simulink model "multi_vehicle"  (R2024a)
settings: Solver=VariableStepAuto  StartTime=0.0  StopTime=600  RelTol=1e-3
settings Model: Creator=sprinkle  LastModifiedBy=Yizhou
settings OptimizationCC: ReuseModelBlockBuffer=off
settings RTWCC: GPUComputeCapability=3.5

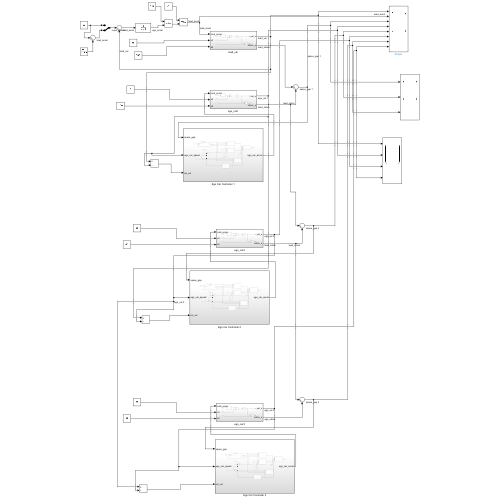
[thumbnail: Simulink's stored preview of the top-level diagram]
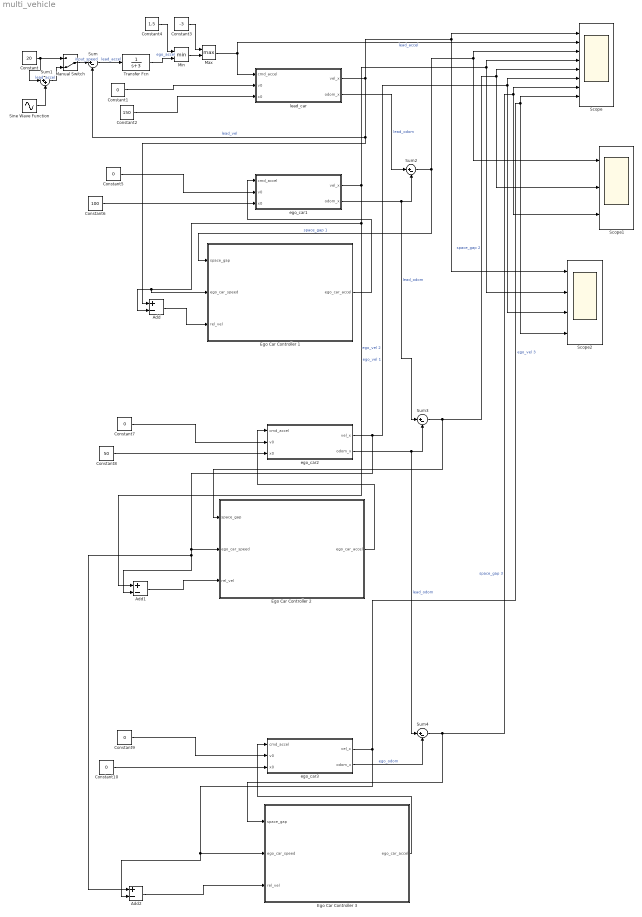
== system multi_vehicle ==
  Add : Sum  Inputs=+-
  Add1 : Sum  Inputs=+-
  Add2 : Sum  Inputs=+-
  Constant : Constant  Value=20
  Constant{1,5,7,9..10} (5 alike) : Constant  Value=0
  Constant2 : Constant  Value=150
  Constant3 : Constant  Value=-3
  Constant4 : Constant  Value=1.5
  Constant6 : Constant  Value=100
  Constant8 : Constant  Value=50
  Ego Car Controller 1 : Subsystem
  Ego Car Controller 2 : Subsystem
  Ego Car Controller 3 : Subsystem
  Manual Switch : ManualSwitch  CurrentSetting=0
  Max : MinMax  Function=max  Inputs=2
  Min : MinMax  Inputs=2
  Scope : Scope  NumInputPorts=8
  Scope1 : Scope  NumInputPorts=3
  Scope2 : Scope  NumInputPorts=4
  Sine Wave Function : Sin  Amplitude=3  Frequency=0.3  SampleTime=0
  Sum{,2..4} (4 alike) : Sum  Inputs=|+-
  Sum1 : Sum  Inputs=|++
  Transfer Fcn : TransferFcn  Denominator=[1 3]
  ego_car1 : Subsystem
  ego_car2 : Subsystem
  ego_car3 : Subsystem
  lead_car : Subsystem
  wires:
  Constant/1 -> Sum1/1, Manual Switch/1
  lead_car/1(vel_x) -> Scope2/1, Scope/1, Add/1, Sum/2  "lead_vel"
  Constant1/1 -> lead_car/2(v0)
  Constant2/1 -> lead_car/3(x0)
  Sum/1 -> Transfer Fcn/1  "lead_accel"
  Manual Switch/1 -> Sum/1  "input_speed"
  Max/1 -> lead_car/1(cmd_accel), Scope/2  "lead_accel"
  Constant4/1 -> Min/1
  Constant3/1 -> Max/1
  Min/1 -> Max/2
  Sine Wave Function/1 -> Sum1/2
  Sum1/1 -> Manual Switch/2  "lead_accel"
  Transfer Fcn/1 -> Min/2  "ego_accel"
  Sum2/1 -> Ego Car Controller 1/1(space_gap), Scope1/1, Scope/3  "space_gap 1"
  lead_car/2(odom_x) -> Sum2/1  "lead_odom"
  ego_car1/1(vel_x) -> Add1/1, Ego Car Controller 1/2(ego_car_speed), Add/2, Scope2/2, Scope/4  "ego_vel 1"
  Ego Car Controller 1/1(ego_car_accel) -> ego_car1/1(cmd_accel)
  Constant5/1 -> ego_car1/2(v0)
  Constant6/1 -> ego_car1/3(x0)
  Constant8/1 -> ego_car2/3(x0)
  Constant7/1 -> ego_car2/2(v0)
  Ego Car Controller 2/1(ego_car_accel) -> ego_car2/1(cmd_accel)
  Sum3/1 -> Ego Car Controller 2/1(space_gap), Scope1/2, Scope/5  "space_gap 2"
  ego_car1/2(odom_x) -> Sum2/2, Sum3/1  "lead_odom"
  Ego Car Controller 3/1(ego_car_accel) -> ego_car3/1(cmd_accel)
  ego_car2/1(vel_x) -> Ego Car Controller 2/2(ego_car_speed), Add1/2, Add2/1, Scope2/3, Scope/6  "ego_vel 2"
  ego_car3/1(vel_x) -> Ego Car Controller 3/2(ego_car_speed), Add2/2, Scope2/4, Scope/8  "ego_vel 3"
  ego_car3/2(odom_x) -> Sum4/2  "ego_odom"
  Constant10/1 -> ego_car3/3(x0)
  Constant9/1 -> ego_car3/2(v0)
  Sum4/1 -> Ego Car Controller 3/1(space_gap), Scope1/3, Scope/7  "space_gap 3"
  ego_car2/2(odom_x) -> Sum4/1, Sum3/2  "lead_odom"
  Add/1 -> Ego Car Controller 1/3(rel_vel)
  Add1/1 -> Ego Car Controller 2/3(rel_vel)
  Add2/1 -> Ego Car Controller 3/3(rel_vel)

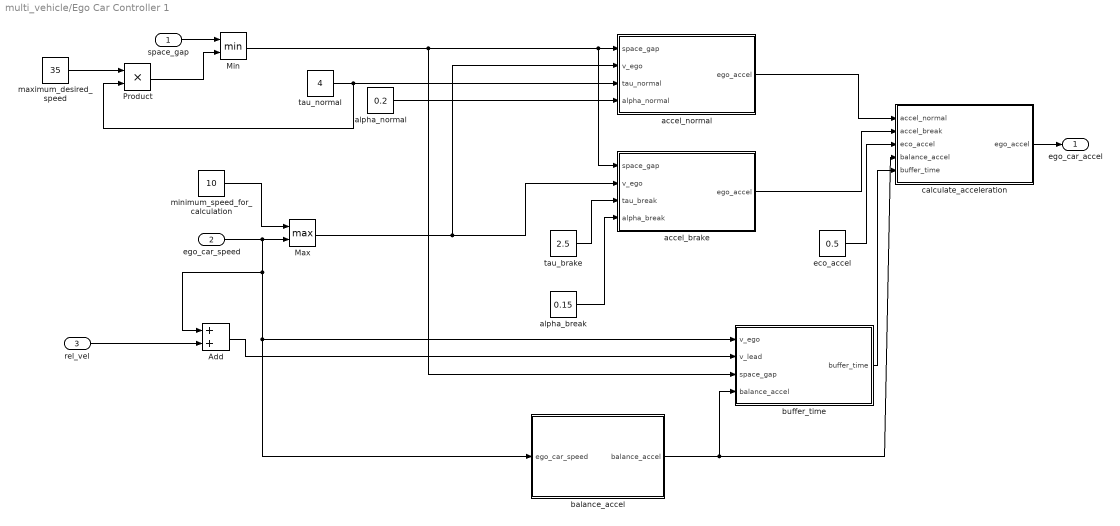
== system multi_vehicle/Ego Car Controller 1 ==
  space_gap : Inport
  ego_car_speed : Inport  Port=2
  rel_vel : Inport  Port=3
  Add : Sum
  Max : MinMax  Function=max  Inputs=2
  Min : MinMax  Inputs=2
  Product : Product
  accel_brake : MATLAB Function  TreatAsAtomicUnit=on
  accel_normal : MATLAB Function  TreatAsAtomicUnit=on
  alpha_break : Constant  Value=0.15
  alpha_normal : Constant  Value=0.2
  balance_accel : MATLAB Function  TreatAsAtomicUnit=on
  buffer_time : MATLAB Function  TreatAsAtomicUnit=on
  calculate_acceleration : MATLAB Function  TreatAsAtomicUnit=on
  eco_accel : Constant  Value=0.5
  maximum_desired_speed : Constant  Value=35
  minimum_speed_for_calculation : Constant  Value=10
  tau_brake : Constant  Value=2.5
  tau_normal : Constant  Value=4
  ego_car_accel : Outport
  wires:
  Max/1 -> accel_normal/2(v_ego), accel_brake/2(v_ego)
  Min/1 -> buffer_time/3(space_gap), accel_normal/1(space_gap), accel_brake/1(space_gap)
  alpha_normal/1 -> accel_normal/4(alpha_normal)
  tau_brake/1 -> accel_brake/3(tau_break)
  alpha_break/1 -> accel_brake/4(alpha_break)
  accel_normal/1(ego_accel) -> calculate_acceleration/1(accel_normal)
  eco_accel/1 -> calculate_acceleration/3(eco_accel)
  balance_accel/1(balance_accel) -> buffer_time/4(balance_accel), calculate_acceleration/4(balance_accel)
  accel_brake/1(ego_accel) -> calculate_acceleration/2(accel_break)
  ego_car_speed/1 -> Add/1, buffer_time/1(v_ego), balance_accel/1(ego_car_speed), Max/2
  minimum_speed_for_calculation/1 -> Max/1
  space_gap/1 -> Min/1
  Product/1 -> Min/2
  calculate_acceleration/1(ego_accel) -> ego_car_accel/1
  tau_normal/1 -> Product/2, accel_normal/3(tau_normal)
  maximum_desired_speed/1 -> Product/1
  rel_vel/1 -> Add/2
  buffer_time/1(buffer_time) -> calculate_acceleration/5(buffer_time)
  Add/1 -> buffer_time/2(v_lead)

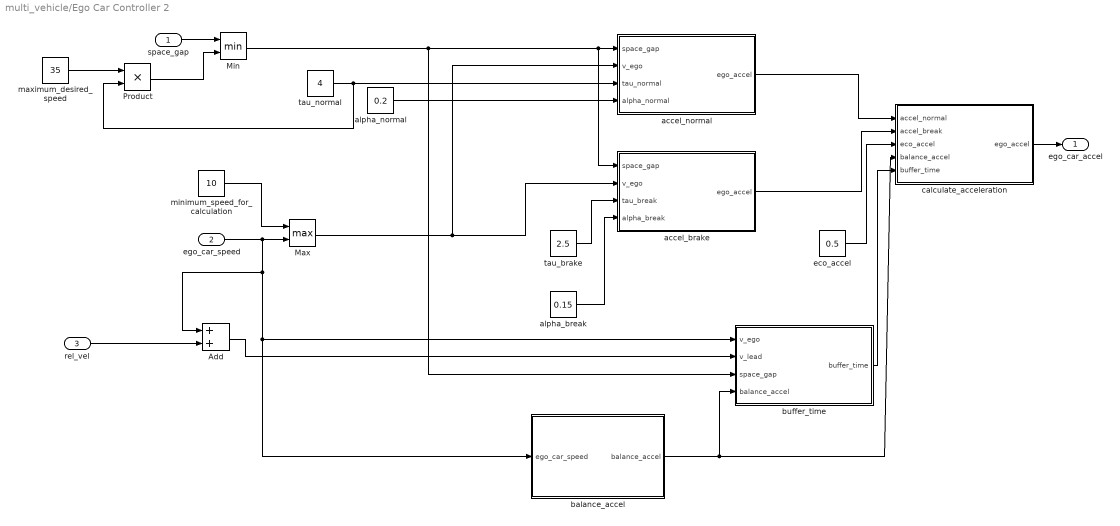
== system multi_vehicle/Ego Car Controller 2 ==
  space_gap : Inport
  ego_car_speed : Inport  Port=2
  rel_vel : Inport  Port=3
  Add : Sum
  Max : MinMax  Function=max  Inputs=2
  Min : MinMax  Inputs=2
  Product : Product
  accel_brake : MATLAB Function  TreatAsAtomicUnit=on
  accel_normal : MATLAB Function  TreatAsAtomicUnit=on
  alpha_break : Constant  Value=0.15
  alpha_normal : Constant  Value=0.2
  balance_accel : MATLAB Function  TreatAsAtomicUnit=on
  buffer_time : MATLAB Function  TreatAsAtomicUnit=on
  calculate_acceleration : MATLAB Function  TreatAsAtomicUnit=on
  eco_accel : Constant  Value=0.5
  maximum_desired_speed : Constant  Value=35
  minimum_speed_for_calculation : Constant  Value=10
  tau_brake : Constant  Value=2.5
  tau_normal : Constant  Value=4
  ego_car_accel : Outport
  wires:
  Max/1 -> accel_normal/2(v_ego), accel_brake/2(v_ego)
  Min/1 -> buffer_time/3(space_gap), accel_normal/1(space_gap), accel_brake/1(space_gap)
  alpha_normal/1 -> accel_normal/4(alpha_normal)
  tau_brake/1 -> accel_brake/3(tau_break)
  alpha_break/1 -> accel_brake/4(alpha_break)
  accel_normal/1(ego_accel) -> calculate_acceleration/1(accel_normal)
  eco_accel/1 -> calculate_acceleration/3(eco_accel)
  balance_accel/1(balance_accel) -> buffer_time/4(balance_accel), calculate_acceleration/4(balance_accel)
  accel_brake/1(ego_accel) -> calculate_acceleration/2(accel_break)
  ego_car_speed/1 -> Add/1, buffer_time/1(v_ego), balance_accel/1(ego_car_speed), Max/2
  minimum_speed_for_calculation/1 -> Max/1
  space_gap/1 -> Min/1
  Product/1 -> Min/2
  calculate_acceleration/1(ego_accel) -> ego_car_accel/1
  tau_normal/1 -> Product/2, accel_normal/3(tau_normal)
  maximum_desired_speed/1 -> Product/1
  rel_vel/1 -> Add/2
  buffer_time/1(buffer_time) -> calculate_acceleration/5(buffer_time)
  Add/1 -> buffer_time/2(v_lead)

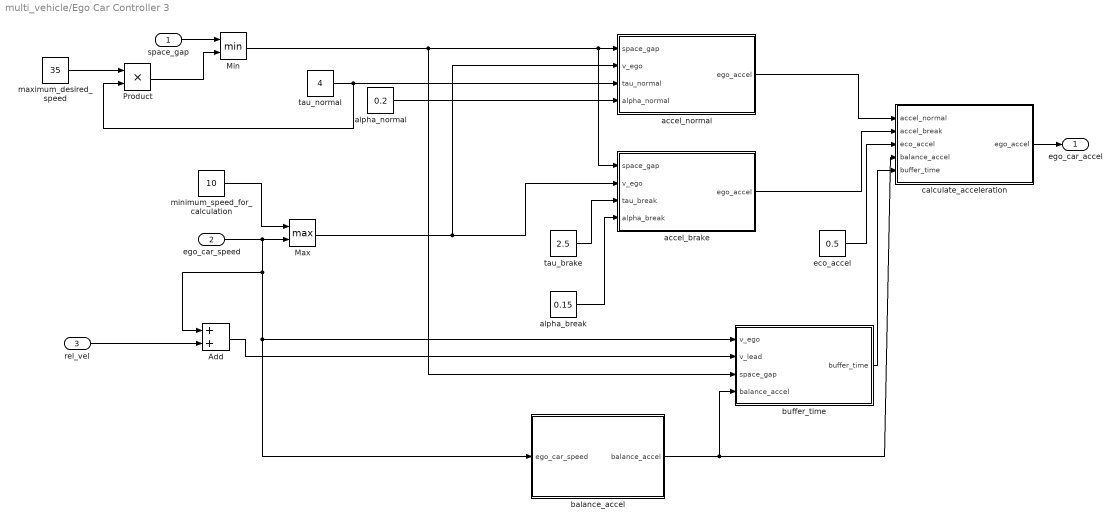
== system multi_vehicle/Ego Car Controller 3 ==
  space_gap : Inport
  ego_car_speed : Inport  Port=2
  rel_vel : Inport  Port=3
  Add : Sum
  Max : MinMax  Function=max  Inputs=2
  Min : MinMax  Inputs=2
  Product : Product
  accel_brake : MATLAB Function  TreatAsAtomicUnit=on
  accel_normal : MATLAB Function  TreatAsAtomicUnit=on
  alpha_break : Constant  Value=0.15
  alpha_normal : Constant  Value=0.2
  balance_accel : MATLAB Function  TreatAsAtomicUnit=on
  buffer_time : MATLAB Function  TreatAsAtomicUnit=on
  calculate_acceleration : MATLAB Function  TreatAsAtomicUnit=on
  eco_accel : Constant  Value=0.5
  maximum_desired_speed : Constant  Value=35
  minimum_speed_for_calculation : Constant  Value=10
  tau_brake : Constant  Value=2.5
  tau_normal : Constant  Value=4
  ego_car_accel : Outport
  wires:
  Max/1 -> accel_normal/2(v_ego), accel_brake/2(v_ego)
  Min/1 -> buffer_time/3(space_gap), accel_normal/1(space_gap), accel_brake/1(space_gap)
  alpha_normal/1 -> accel_normal/4(alpha_normal)
  tau_brake/1 -> accel_brake/3(tau_break)
  alpha_break/1 -> accel_brake/4(alpha_break)
  accel_normal/1(ego_accel) -> calculate_acceleration/1(accel_normal)
  eco_accel/1 -> calculate_acceleration/3(eco_accel)
  balance_accel/1(balance_accel) -> buffer_time/4(balance_accel), calculate_acceleration/4(balance_accel)
  accel_brake/1(ego_accel) -> calculate_acceleration/2(accel_break)
  ego_car_speed/1 -> Add/1, buffer_time/1(v_ego), balance_accel/1(ego_car_speed), Max/2
  minimum_speed_for_calculation/1 -> Max/1
  space_gap/1 -> Min/1
  Product/1 -> Min/2
  calculate_acceleration/1(ego_accel) -> ego_car_accel/1
  tau_normal/1 -> Product/2, accel_normal/3(tau_normal)
  maximum_desired_speed/1 -> Product/1
  rel_vel/1 -> Add/2
  buffer_time/1(buffer_time) -> calculate_acceleration/5(buffer_time)
  Add/1 -> buffer_time/2(v_lead)

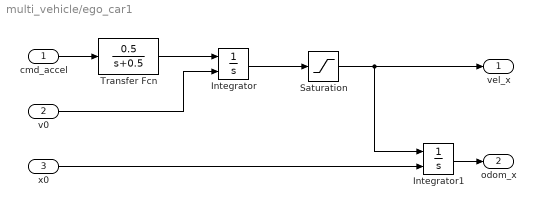
== system multi_vehicle/ego_car1 ==
  cmd_accel : Inport
  v0 : Inport  Port=2
  x0 : Inport  Port=3
  Integrator : Integrator  InitialConditionSource=external
  Integrator1 : Integrator  InitialConditionSource=external
  Saturation : Saturate  UpperLimit=80  LowerLimit=0
  Transfer Fcn : TransferFcn  Numerator=[0.5]  Denominator=[1 0.5]
  vel_x : Outport
  odom_x : Outport  Port=2
  wires:
  v0/1 -> Integrator/2
  cmd_accel/1 -> Transfer Fcn/1
  Transfer Fcn/1 -> Integrator/1
  Integrator1/1 -> odom_x/1
  Integrator/1 -> Saturation/1
  x0/1 -> Integrator1/2
  Saturation/1 -> vel_x/1, Integrator1/1

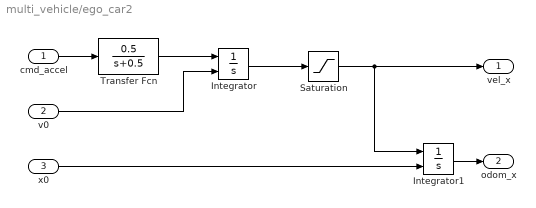
== system multi_vehicle/ego_car2 ==
  cmd_accel : Inport
  v0 : Inport  Port=2
  x0 : Inport  Port=3
  Integrator : Integrator  InitialConditionSource=external
  Integrator1 : Integrator  InitialConditionSource=external
  Saturation : Saturate  UpperLimit=80  LowerLimit=0
  Transfer Fcn : TransferFcn  Numerator=[0.5]  Denominator=[1 0.5]
  vel_x : Outport
  odom_x : Outport  Port=2
  wires:
  v0/1 -> Integrator/2
  cmd_accel/1 -> Transfer Fcn/1
  Transfer Fcn/1 -> Integrator/1
  Integrator1/1 -> odom_x/1
  Integrator/1 -> Saturation/1
  x0/1 -> Integrator1/2
  Saturation/1 -> vel_x/1, Integrator1/1

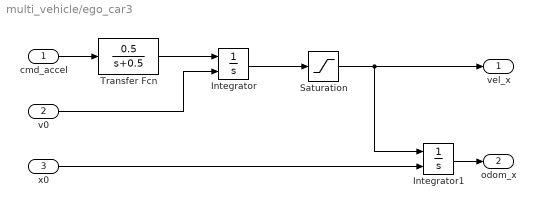
== system multi_vehicle/ego_car3 ==
  cmd_accel : Inport
  v0 : Inport  Port=2
  x0 : Inport  Port=3
  Integrator : Integrator  InitialConditionSource=external
  Integrator1 : Integrator  InitialConditionSource=external
  Saturation : Saturate  UpperLimit=80  LowerLimit=0
  Transfer Fcn : TransferFcn  Numerator=[0.5]  Denominator=[1 0.5]
  vel_x : Outport
  odom_x : Outport  Port=2
  wires:
  v0/1 -> Integrator/2
  cmd_accel/1 -> Transfer Fcn/1
  Transfer Fcn/1 -> Integrator/1
  Integrator1/1 -> odom_x/1
  Integrator/1 -> Saturation/1
  x0/1 -> Integrator1/2
  Saturation/1 -> vel_x/1, Integrator1/1

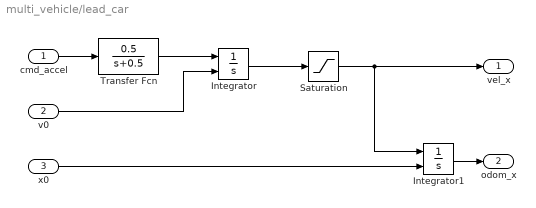
== system multi_vehicle/lead_car ==
  cmd_accel : Inport
  v0 : Inport  Port=2
  x0 : Inport  Port=3
  Integrator : Integrator  InitialConditionSource=external
  Integrator1 : Integrator  InitialConditionSource=external
  Saturation : Saturate  UpperLimit=80  LowerLimit=0
  Transfer Fcn : TransferFcn  Numerator=[0.5]  Denominator=[1 0.5]
  vel_x : Outport
  odom_x : Outport  Port=2
  wires:
  v0/1 -> Integrator/2
  cmd_accel/1 -> Transfer Fcn/1
  Transfer Fcn/1 -> Integrator/1
  Integrator1/1 -> odom_x/1
  Integrator/1 -> Saturation/1
  x0/1 -> Integrator1/2
  Saturation/1 -> vel_x/1, Integrator1/1

== matlab function multi_vehicle/Ego Car Controller 3/accel_brake ==
  data: space_gap input; ego_accel output; v_ego input; tau_break input; alpha_break input
function ego_accel = fcn(space_gap, v_ego, tau_break, alpha_break)

ego_accel = (alpha_break*(space_gap - tau_break * v_ego));
ego_accel = min(ego_accel, 1.5);
ego_accel = max(ego_accel, -3);

== matlab function multi_vehicle/Ego Car Controller 3/accel_normal ==
  data: space_gap input; v_ego input; tau_normal input; alpha_normal input; ego_accel output
function ego_accel = fcn(space_gap, v_ego, tau_normal, alpha_normal)

ego_accel = (alpha_normal * (space_gap - tau_normal * v_ego));
ego_accel = min(ego_accel, 1.5);
ego_accel = max(ego_accel, -3);

== matlab function multi_vehicle/Ego Car Controller 1/accel_normal ==
  data: space_gap input; v_ego input; tau_normal input; alpha_normal input; ego_accel output
function ego_accel = fcn(space_gap, v_ego, tau_normal, alpha_normal)

ego_accel = (alpha_normal * (space_gap - tau_normal * v_ego));
ego_accel = min(ego_accel, 1.5);
ego_accel = max(ego_accel, -3);

== matlab function multi_vehicle/Ego Car Controller 3/balance_accel ==
  data: ego_car_speed input; balance_accel output
function balance_accel = fcn(ego_car_speed)

balance_accel = -0.00021453 * (ego_car_speed * ego_car_speed) - 0.14715;

== matlab function multi_vehicle/Ego Car Controller 3/buffer_time ==
  data: v_ego input; v_lead input; space_gap input; buffer_time output; balance_accel input
function buffer_time = fcn(v_ego, v_lead, space_gap, balance_accel)

% Calculate distance needed for ego car to match lead_car speed to brake at
% balance_accel
brake_dist = (v_ego+v_lead)/2*(v_ego - v_lead)/(0-balance_accel);
% Calculate time needed, and safe_dist should be maintained after coasting
buffer_time=(space_gap-brake_dist)/v_ego;
% let maximum speed difference be 3m/s
if (v_ego-v_lead) > 3
    buffer_time = 0;
end

== matlab function multi_vehicle/Ego Car Controller 3/calculate_acceleration ==
  data: accel_normal input; ego_accel output; accel_break input; eco_accel input; balance_accel input; buffer_time input
function ego_accel = fcn(accel_normal, accel_break, eco_accel, balance_accel, buffer_time) 
    
    if buffer_time < 10
        ego_accel = min(accel_break,balance_accel);
    elseif accel_normal > 0
        ego_accel = min(accel_normal, eco_accel);
    elseif accel_break > 0
    
        ego_accel = max(accel_normal, balance_accel);
    else
        ego_accel = accel_break;
    end


    if ego_accel > 1.5
        ego_accel = 1.5;
    end
    if ego_accel < -3
        ego_accel = -3;
    end

end

== matlab function multi_vehicle/Ego Car Controller 1/accel_brake ==
  data: space_gap input; ego_accel output; v_ego input; tau_break input; alpha_break input
function ego_accel = fcn(space_gap, v_ego, tau_break, alpha_break)

ego_accel = (alpha_break*(space_gap - tau_break * v_ego));
ego_accel = min(ego_accel, 1.5);
ego_accel = max(ego_accel, -3);

== matlab function multi_vehicle/Ego Car Controller 1/calculate_acceleration ==
  data: accel_normal input; ego_accel output; accel_break input; eco_accel input; balance_accel input; buffer_time input
function ego_accel = fcn(accel_normal, accel_break, eco_accel, balance_accel, buffer_time) 
    
    if buffer_time < 10
        ego_accel = min(accel_break,balance_accel);
    elseif accel_normal > 0
        ego_accel = min(accel_normal, eco_accel);
    elseif accel_break > 0
    
        ego_accel = max(accel_normal, balance_accel);
    else
        ego_accel = accel_break;
    end


    if ego_accel > 1.5
        ego_accel = 1.5;
    end
    if ego_accel < -3
        ego_accel = -3;
    end

end

== matlab function multi_vehicle/Ego Car Controller 1/balance_accel ==
  data: ego_car_speed input; balance_accel output
function balance_accel = fcn(ego_car_speed)

balance_accel = -0.00021453 * (ego_car_speed * ego_car_speed) - 0.14715;

== matlab function multi_vehicle/Ego Car Controller 1/buffer_time ==
  data: v_ego input; v_lead input; space_gap input; buffer_time output; balance_accel input
function buffer_time = fcn(v_ego, v_lead, space_gap, balance_accel)

% Calculate distance needed for ego car to match lead_car speed to brake at
% balance_accel
brake_dist = (v_ego+v_lead)/2*(v_ego - v_lead)/(0-balance_accel);
% Calculate time needed, and safe_dist should be maintained after coasting
buffer_time=(space_gap-brake_dist)/v_ego;
% let maximum speed difference be 3m/s
if (v_ego-v_lead) > 3
    buffer_time = 0;
end

== matlab function multi_vehicle/Ego Car Controller 2/accel_brake ==
  data: space_gap input; ego_accel output; v_ego input; tau_break input; alpha_break input
function ego_accel = fcn(space_gap, v_ego, tau_break, alpha_break)

ego_accel = (alpha_break*(space_gap - tau_break * v_ego));
ego_accel = min(ego_accel, 1.5);
ego_accel = max(ego_accel, -3);

== matlab function multi_vehicle/Ego Car Controller 2/accel_normal ==
  data: space_gap input; v_ego input; tau_normal input; alpha_normal input; ego_accel output
function ego_accel = fcn(space_gap, v_ego, tau_normal, alpha_normal)

ego_accel = (alpha_normal * (space_gap - tau_normal * v_ego));
ego_accel = min(ego_accel, 1.5);
ego_accel = max(ego_accel, -3);

== matlab function multi_vehicle/Ego Car Controller 2/balance_accel ==
  data: ego_car_speed input; balance_accel output
function balance_accel = fcn(ego_car_speed)

balance_accel = -0.00021453 * (ego_car_speed * ego_car_speed) - 0.14715;

== matlab function multi_vehicle/Ego Car Controller 2/buffer_time ==
  data: v_ego input; v_lead input; space_gap input; buffer_time output; balance_accel input
function buffer_time = fcn(v_ego, v_lead, space_gap, balance_accel)

% Calculate distance needed for ego car to match lead_car speed to brake at
% balance_accel
brake_dist = (v_ego+v_lead)/2*(v_ego - v_lead)/(0-balance_accel);
% Calculate time needed, and safe_dist should be maintained after coasting
buffer_time=(space_gap-brake_dist)/v_ego;
% let maximum speed difference be 3m/s
if (v_ego-v_lead) > 3
    buffer_time = 0;
end

== matlab function multi_vehicle/Ego Car Controller 2/calculate_acceleration ==
  data: accel_normal input; ego_accel output; accel_break input; eco_accel input; balance_accel input; buffer_time input
function ego_accel = fcn(accel_normal, accel_break, eco_accel, balance_accel, buffer_time) 
    
    if buffer_time < 10
        ego_accel = min(accel_break,balance_accel);
    elseif accel_normal > 0
        ego_accel = min(accel_normal, eco_accel);
    elseif accel_break > 0
    
        ego_accel = max(accel_normal, balance_accel);
    else
        ego_accel = accel_break;
    end


    if ego_accel > 1.5
        ego_accel = 1.5;
    end
    if ego_accel < -3
        ego_accel = -3;
    end

end
